simulink model "sys10m_pss"  (Simulink 8.7)
settings: Solver=ode3  StartTime=0.0  StopTime=10  FixedStep=1e-2  MaxStep=1e-2  RelTol=1e-5
values from neighbouring files (symbols this model uses):
  Kpss1 = KG1*T11*T13/(T12*T14)    [initSSA.m]    (also in pss_objf.m)
  Kpss10 = KG10*T101*T103/(T102*T104)    [initSSA.m]    (also in pss_objf.m)
  Kpss3 = KG3*T31*T33/(T32*T34)    [initSSA.m]    (also in pss_objf.m)
  Kpss4 = KG4*T41*T43/(T42*T44)    [initSSA.m]    (also in pss_objf.m)
  Kpss5 = KG5*T51*T53/(T52*T54)    [initSSA.m]    (also in pss_objf.m)
  Kpss6 = KG6*T61*T63/(T62*T64)    [initSSA.m]    (also in pss_objf.m)
  Kpss7 = KG7*T71*T73/(T72*T74)    [initSSA.m]    (also in pss_objf.m)
  Kpss8 = KG8*T81*T83/(T82*T84)    [initSSA.m]    (also in pss_objf.m)
  Kpss9 = KG9*T91*T93/(T92*T94)    [initSSA.m]    (also in pss_objf.m)
  T101 = x(42)    [initSSA.m]    (also in pss_objf.m)
  T102 = x(43)    [initSSA.m]    (also in pss_objf.m)
  T103 = x(44)    [initSSA.m]    (also in pss_objf.m)
  T104 = x(45)    [initSSA.m]    (also in pss_objf.m)
  T11 = x(10)    [initSSA.m]    (also in pss_objf.m)
  T12 = x(11)    [initSSA.m]    (also in pss_objf.m)
  T13 = x(12)    [initSSA.m]    (also in pss_objf.m)
  T14 = x(13)    [initSSA.m]    (also in pss_objf.m)
  T31 = x(14)    [initSSA.m]    (also in pss_objf.m)
  T32 = x(15)    [initSSA.m]    (also in pss_objf.m)
  T33 = x(16)    [initSSA.m]    (also in pss_objf.m)
  T34 = x(17)    [initSSA.m]    (also in pss_objf.m)
  T41 = x(18)    [initSSA.m]    (also in pss_objf.m)
  T42 = x(19)    [initSSA.m]    (also in pss_objf.m)
  T43 = x(20)    [initSSA.m]    (also in pss_objf.m)
  T44 = x(21)    [initSSA.m]    (also in pss_objf.m)
  T51 = x(22)    [initSSA.m]    (also in pss_objf.m)
  T52 = x(23)    [initSSA.m]    (also in pss_objf.m)
  T53 = x(24)    [initSSA.m]    (also in pss_objf.m)
  T54 = x(25)    [initSSA.m]    (also in pss_objf.m)
  T61 = x(26)    [initSSA.m]    (also in pss_objf.m)
  T62 = x(27)    [initSSA.m]    (also in pss_objf.m)
  T63 = x(28)    [initSSA.m]    (also in pss_objf.m)
  T64 = x(29)    [initSSA.m]    (also in pss_objf.m)
  T71 = x(30)    [initSSA.m]    (also in pss_objf.m)
  T72 = x(31)    [initSSA.m]    (also in pss_objf.m)
  T73 = x(32)    [initSSA.m]    (also in pss_objf.m)
  T74 = x(33)    [initSSA.m]    (also in pss_objf.m)
  T81 = x(34)    [initSSA.m]    (also in pss_objf.m)
  T82 = x(35)    [initSSA.m]    (also in pss_objf.m)
  T83 = x(36)    [initSSA.m]    (also in pss_objf.m)
  T84 = x(37)    [initSSA.m]    (also in pss_objf.m)
  T91 = x(38)    [initSSA.m]    (also in pss_objf.m)
  T92 = x(39)    [initSSA.m]    (also in pss_objf.m)
  T93 = x(40)    [initSSA.m]    (also in pss_objf.m)
  T94 = x(41)    [initSSA.m]    (also in pss_objf.m)
  Tw = 10    [initSSA.m]    (also in pss_objf.m)
undefined symbols (not defined in the file or in its folder): D, delta0, Efd0, Epd0, Epq0, event, fYred, KA, M, m, small_d, TA, Tpd0, Tpq0, Vref1, ws, XXdpd, XXpdq, XXqpq, Yred, Zdq
libraries: powerlib_extras x2
settings Model: Creator=hbeiran  LastModifiedBy=EBUKA
settings SolverCC: AlgebraicLoopSolver=LineSearch
settings DataIOCC: LimitDataPoints=off  SignalLoggingSaveFormat=ModelDataLogs
settings OptimizationCC: DefaultParameterBehavior=Inlined  BufferReuse=off  ExpressionDepthLimit=2147483647
settings DebuggingCC: AlgebraicLoopMsg=none  SolverPrmCheckMsg=warning  FcnCallInpInsideContextMsg=UseLocalSettings  StateNameClashWarn=warning  InitInArrayFormatMsg=none
settings SFSimCC: SimParseCustomCode=off
settings GRTTargetCC: CombineOutputUpdateFcns=off  GRTInterface=on
settings ConfigurationSet: Description=SimMechanics 2G

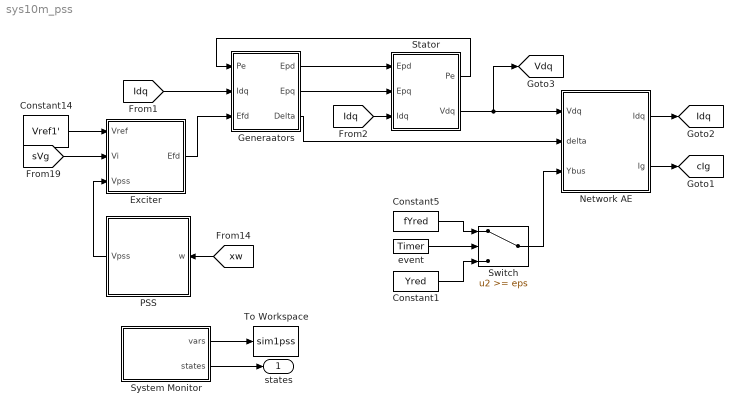
== system sys10m_pss ==
  Constant1 : Constant  Value=Yred  VectorParams1D=off
  Constant14 : Constant  Value=Vref1'  VectorParams1D=off
  Constant5 : Constant  Value=fYred  VectorParams1D=off
  Exciter : Subsystem
  Generaators : Subsystem
  Network AE : MATLAB Function  TreatAsAtomicUnit=on
  PSS : Subsystem
  Stator : Subsystem
  Switch : Switch  Threshold=eps
  System Monitor : Subsystem
  To Workspace : ToWorkspace  VariableName=sim1pss  SaveFormat=Structure With Time  SampleTime=-1
  event : powerlib_extras/Control  Blocks/Timer  t=event(1,:)  e=event(2,:)
  states : Outport
  tag scope: Idq=global, Vdq=global, cIg=global
  wires:
  Exciter/1(Efd) -> Generaators/3(Efd)
  Constant14/1 -> Exciter/1(Vref)
  [Idq] -> Generaators/2(Idq)
  Network AE/1(Idq) -> [Idq]
  event/1 -> Switch/2
  Constant5/1 -> Switch/1
  Constant1/1 -> Switch/3
  Switch/1 -> Network AE/3(Ybus)
  System Monitor/1(vars) -> To Workspace/1
  System Monitor/2(states) -> states/1
  Generaators/3(Delta) -> Network AE/2(delta)
  Network AE/2(Ig) -> [cIg]
  Stator/2(Vdq) -> Network AE/1(Vdq), [Vdq]
  [Idq] -> Stator/3(Idq)
  Generaators/1(Epd) -> Stator/1(Epd)
  Generaators/2(Epq) -> Stator/2(Epq)
  Stator/1(Pe) -> Generaators/1(Pe)
  [sVg] -> Exciter/2(Vi)
  PSS/1(Vpss) -> Exciter/3(Vpss)
  [xw] -> PSS/1(w)

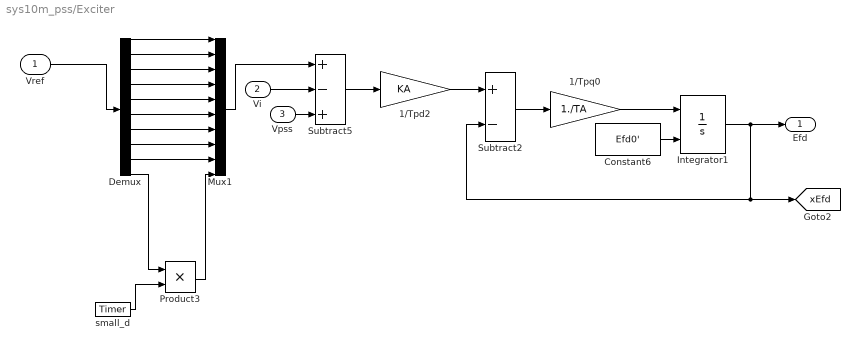
== system sys10m_pss/Exciter ==
  Vref : Inport
  Vi : Inport  Port=2
  Vpss : Inport  Port=3
  1/Tpd2 : Gain  Gain=KA
  1/Tpq0 : Gain  Gain=1./TA
  Constant6 : Constant  Value=Efd0'  VectorParams1D=off
  Demux : Demux  Outputs=10
  Integrator1 : Integrator  InitialConditionSource=external
  Mux1 : Mux  Inputs=10
  Product3 : Product  RndMeth=Zero
  Subtract2 : Sum  Inputs=+-
  Subtract5 : Sum  Inputs=+-+
  small_d : powerlib_extras/Control  Blocks/Timer  t=small_d(1,:)  e=small_d(2,:)
  Efd : Outport
  tag scope: xEfd=global
  wires:
  Constant6/1 -> Integrator1/2
  Subtract2/1 -> 1/Tpq0/1
  1/Tpq0/1 -> Integrator1/1
  Integrator1/1 -> Efd/1, Subtract2/2, [xEfd]
  Vi/1 -> Subtract5/2
  Subtract5/1 -> 1/Tpd2/1
  1/Tpd2/1 -> Subtract2/1
  Demux/1 -> Mux1/1
  Demux/2 -> Mux1/2
  small_d/1 -> Product3/2
  Mux1/1 -> Subtract5/1
  Vref/1 -> Demux/1
  Vpss/1 -> Subtract5/3
  Demux/3 -> Mux1/3
  Demux/4 -> Mux1/4
  Demux/5 -> Mux1/5
  Demux/6 -> Mux1/6
  Demux/7 -> Mux1/7
  Demux/8 -> Mux1/8
  Demux/9 -> Mux1/9
  Demux/10 -> Product3/1
  Product3/1 -> Mux1/10

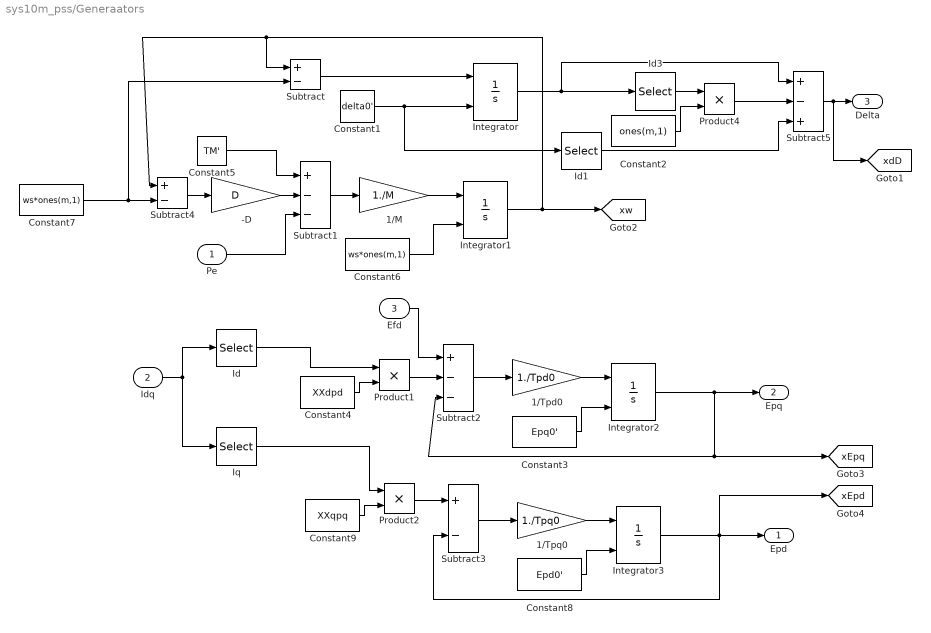
== system sys10m_pss/Generaators ==
  Pe : Inport
  Idq : Inport  Port=2
  Efd : Inport  Port=3
  -D : Gain  Gain=D
  1/M : Gain  Gain=1./M
  1/Tpd0 : Gain  Gain=1./Tpd0
  1/Tpq0 : Gain  Gain=1./Tpq0
  Constant1 : Constant  Value=delta0'  VectorParams1D=off
  Constant2 : Constant  Value=ones(m,1)  VectorParams1D=off
  Constant3 : Constant  Value=Epq0'  VectorParams1D=off
  Constant4 : Constant  Value=XXdpd  VectorParams1D=off
  Constant5 : Constant  Value=TM'  VectorParams1D=off
  Constant6 : Constant  Value=ws*ones(m,1)  VectorParams1D=off
  Constant7 : Constant  Value=ws*ones(m,1)  VectorParams1D=off
  Constant8 : Constant  Value=Epd0'  VectorParams1D=off
  Constant9 : Constant  Value=XXqpq  VectorParams1D=off
  Id : Selector  InputPortWidth=2*m  IndexOptions=Index vector (dialog)  Indices=[1:m]  OutputSizes=1
  Id1 : Selector  InputPortWidth=m  IndexOptions=Index vector (dialog)  Indices=[1]  OutputSizes=1
  Id3 : Selector  InputPortWidth=m  IndexOptions=Index vector (dialog)  Indices=[1]  OutputSizes=1
  Integrator{,1..3} (4 alike) : Integrator  InitialConditionSource=external
  Iq : Selector  InputPortWidth=2*m  IndexOptions=Index vector (dialog)  Indices=[m+1:2*m]  OutputSizes=1
  Product1 : Product  RndMeth=Zero
  Product2 : Product  RndMeth=Zero
  Product4 : Product  RndMeth=Zero
  Subtract : Sum  Inputs=+-
  Subtract1 : Sum  Inputs=+--
  Subtract2 : Sum  Inputs=+--
  Subtract3 : Sum  Inputs=+-
  Subtract4 : Sum  Inputs=+-
  Subtract5 : Sum  Inputs=+-+
  Epd : Outport
  Epq : Outport  Port=2
  Delta : Outport  Port=3
  tag scope: xEpd=global, xEpq=global, xdD=global, xw=global
  wires:
  Subtract/1 -> Integrator/1
  Constant5/1 -> Subtract1/1
  Subtract1/1 -> 1/M/1
  1/M/1 -> Integrator1/1
  Constant6/1 -> Integrator1/2
  -D/1 -> Subtract1/2
  Constant3/1 -> Integrator2/2
  Subtract2/1 -> 1/Tpd0/1
  Integrator2/1 -> Epq/1, Subtract2/3, [xEpq]
  Product1/1 -> Subtract2/2
  Constant4/1 -> Product1/2
  1/Tpd0/1 -> Integrator2/1
  Constant8/1 -> Integrator3/2
  Subtract3/1 -> 1/Tpq0/1
  Integrator3/1 -> Epd/1, [xEpd], Subtract3/2
  Constant9/1 -> Product2/2
  1/Tpq0/1 -> Integrator3/1
  Product2/1 -> Subtract3/1
  Efd/1 -> Subtract2/1
  Integrator1/1 -> [xw], Subtract/1, Subtract4/1
  Id/1 -> Product1/1
  Idq/1 -> Id/1, Iq/1
  Iq/1 -> Product2/1
  Pe/1 -> Subtract1/3
  Subtract4/1 -> -D/1
  Constant7/1 -> Subtract4/2, Subtract/2
  Subtract5/1 -> Delta/1, [xdD]
  Constant1/1 -> Integrator/2, Id1/1
  Integrator/1 -> Subtract5/1, Id3/1
  Id3/1 -> Product4/1
  Constant2/1 -> Product4/2
  Product4/1 -> Subtract5/2
  Id1/1 -> Subtract5/3

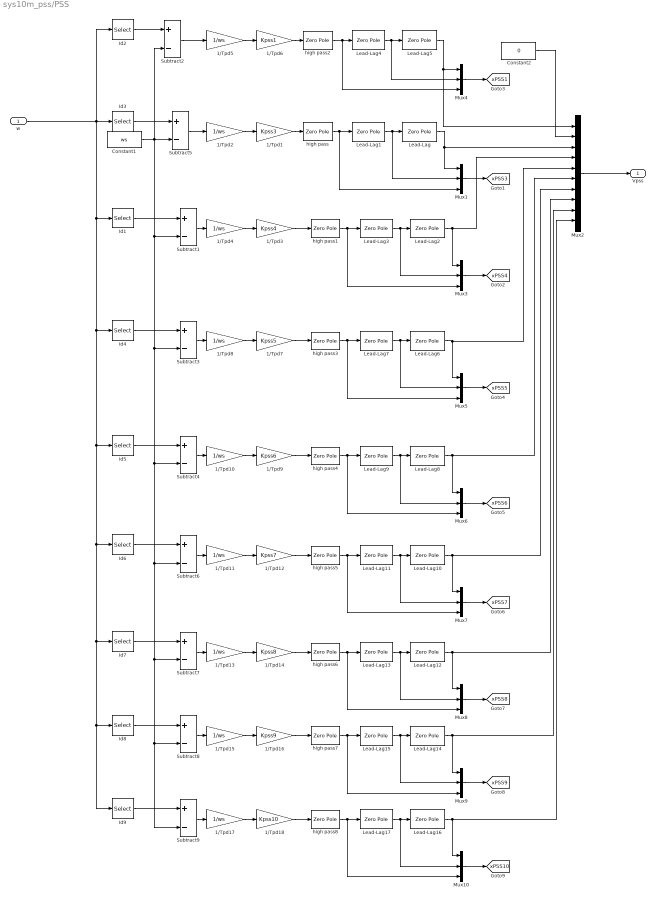
== system sys10m_pss/PSS ==
  w : Inport
  1/Tpd1 : Gain  Gain=Kpss3
  1/Tpd{2,4..5,8,10..11,13,15,17} (9 alike) : Gain  Gain=1/ws
  1/Tpd12 : Gain  Gain=Kpss7
  1/Tpd14 : Gain  Gain=Kpss8
  1/Tpd16 : Gain  Gain=Kpss9
  1/Tpd18 : Gain  Gain=Kpss10
  1/Tpd3 : Gain  Gain=Kpss4
  1/Tpd6 : Gain  Gain=Kpss1
  1/Tpd7 : Gain  Gain=Kpss5
  1/Tpd9 : Gain  Gain=Kpss6
  Constant1 : Constant  Value=ws  VectorParams1D=off
  Constant2 : Constant  Value=0  VectorParams1D=off
  Id1 : Selector  InputPortWidth=m  IndexOptions=Index vector (dialog)  Indices=[4]  OutputSizes=1
  Id2 : Selector  InputPortWidth=m  IndexOptions=Index vector (dialog)  Indices=[1]  OutputSizes=1
  Id3 : Selector  InputPortWidth=m  IndexOptions=Index vector (dialog)  Indices=[3]  OutputSizes=1
  Id4 : Selector  InputPortWidth=m  IndexOptions=Index vector (dialog)  Indices=[5]  OutputSizes=1
  Id5 : Selector  InputPortWidth=m  IndexOptions=Index vector (dialog)  Indices=[6]  OutputSizes=1
  Id6 : Selector  InputPortWidth=m  IndexOptions=Index vector (dialog)  Indices=[7]  OutputSizes=1
  Id7 : Selector  InputPortWidth=m  IndexOptions=Index vector (dialog)  Indices=[8]  OutputSizes=1
  Id8 : Selector  InputPortWidth=m  IndexOptions=Index vector (dialog)  Indices=[9]  OutputSizes=1
  Id9 : Selector  InputPortWidth=m  IndexOptions=Index vector (dialog)  Indices=[10]  OutputSizes=1
  Lead-Lag : ZeroPole  Zeros=[-1/T33]  Poles=[-1/T34]
  Lead-Lag1 : ZeroPole  Zeros=[-1/T31]  Poles=[-1/T32]
  Lead-Lag10 : ZeroPole  Zeros=[-1/T73]  Poles=[-1/T74]
  Lead-Lag11 : ZeroPole  Zeros=[-1/T71]  Poles=[-1/T72]
  Lead-Lag12 : ZeroPole  Zeros=[-1/T83]  Poles=[-1/T84]
  Lead-Lag13 : ZeroPole  Zeros=[-1/T81]  Poles=[-1/T82]
  Lead-Lag14 : ZeroPole  Zeros=[-1/T93]  Poles=[-1/T94]
  Lead-Lag15 : ZeroPole  Zeros=[-1/T91]  Poles=[-1/T92]
  Lead-Lag16 : ZeroPole  Zeros=[-1/T103]  Poles=[-1/T104]
  Lead-Lag17 : ZeroPole  Zeros=[-1/T101]  Poles=[-1/T102]
  Lead-Lag2 : ZeroPole  Zeros=[-1/T43]  Poles=[-1/T44]
  Lead-Lag3 : ZeroPole  Zeros=[-1/T41]  Poles=[-1/T42]
  Lead-Lag4 : ZeroPole  Zeros=[-1/T11]  Poles=[-1/T12]
  Lead-Lag5 : ZeroPole  Zeros=[-1/T13]  Poles=[-1/T14]
  Lead-Lag6 : ZeroPole  Zeros=[-1/T53]  Poles=[-1/T54]
  Lead-Lag7 : ZeroPole  Zeros=[-1/T51]  Poles=[-1/T52]
  Lead-Lag8 : ZeroPole  Zeros=[-1/T63]  Poles=[-1/T64]
  Lead-Lag9 : ZeroPole  Zeros=[-1/T61]  Poles=[-1/T62]
  Mux{1,3..10} (9 alike) : Mux  Inputs=3
  Mux2 : Mux  Inputs=10
  Subtract{1..9} (9 alike) : Sum  Inputs=+-
  high pass{,1..8} (9 alike) : ZeroPole  Zeros=[0]  Poles=[-1/Tw]
  Vpss : Outport
  tag scope: xPSS10=global, xPSS1=global, xPSS3=global, xPSS4=global, xPSS5=global, xPSS6=global, xPSS7=global, xPSS8=global, xPSS9=global
  wires:
  Subtract5/1 -> 1/Tpd2/1
  1/Tpd1/1 -> high pass/1
  Lead-Lag/1 -> Mux2/3, Mux1/1
  high pass/1 -> Lead-Lag1/1, Mux1/3
  Lead-Lag1/1 -> Lead-Lag/1, Mux1/2
  Mux1/1 -> [xPSS3]
  1/Tpd2/1 -> 1/Tpd1/1
  Mux2/1 -> Vpss/1
  Id3/1 -> Subtract5/1
  Subtract1/1 -> 1/Tpd4/1
  1/Tpd3/1 -> high pass1/1
  Lead-Lag2/1 -> Mux2/4, Mux3/1
  high pass1/1 -> Mux3/3, Lead-Lag3/1
  Lead-Lag3/1 -> Mux3/2, Lead-Lag2/1
  Mux3/1 -> [xPSS4]
  1/Tpd4/1 -> 1/Tpd3/1
  Id1/1 -> Subtract1/1
  Id2/1 -> Subtract2/1
  Subtract2/1 -> 1/Tpd5/1
  1/Tpd5/1 -> 1/Tpd6/1
  1/Tpd6/1 -> high pass2/1
  high pass2/1 -> Mux4/3, Lead-Lag4/1
  Lead-Lag4/1 -> Mux4/2, Lead-Lag5/1
  Lead-Lag5/1 -> Mux2/1, Mux4/1
  Mux4/1 -> [xPSS1]
  Subtract3/1 -> 1/Tpd8/1
  1/Tpd7/1 -> high pass3/1
  Lead-Lag6/1 -> Mux2/5, Mux5/1
  high pass3/1 -> Lead-Lag7/1, Mux5/3
  Lead-Lag7/1 -> Lead-Lag6/1, Mux5/2
  Mux5/1 -> [xPSS5]
  1/Tpd8/1 -> 1/Tpd7/1
  Id4/1 -> Subtract3/1
  w/1 -> Id2/1, Id3/1, Id6/1, Id8/1, Id9/1, Id7/1, Id5/1, Id4/1, Id1/1
  Subtract4/1 -> 1/Tpd10/1
  1/Tpd9/1 -> high pass4/1
  high pass4/1 -> Mux6/3, Lead-Lag9/1
  Lead-Lag9/1 -> Mux6/2, Lead-Lag8/1
  Mux6/1 -> [xPSS6]
  1/Tpd10/1 -> 1/Tpd9/1
  Id5/1 -> Subtract4/1
  Subtract6/1 -> 1/Tpd11/1
  1/Tpd12/1 -> high pass5/1
  high pass5/1 -> Lead-Lag11/1, Mux7/3
  Lead-Lag11/1 -> Lead-Lag10/1, Mux7/2
  Mux7/1 -> [xPSS7]
  1/Tpd11/1 -> 1/Tpd12/1
  Id6/1 -> Subtract6/1
  Subtract7/1 -> 1/Tpd13/1
  1/Tpd14/1 -> high pass6/1
  high pass6/1 -> Mux8/3, Lead-Lag13/1
  Lead-Lag13/1 -> Mux8/2, Lead-Lag12/1
  Mux8/1 -> [xPSS8]
  1/Tpd13/1 -> 1/Tpd14/1
  Id7/1 -> Subtract7/1
  Lead-Lag8/1 -> Mux2/6, Mux6/1
  Lead-Lag10/1 -> Mux2/7, Mux7/1
  Lead-Lag12/1 -> Mux2/8, Mux8/1
  Subtract8/1 -> 1/Tpd15/1
  1/Tpd16/1 -> high pass7/1
  high pass7/1 -> Lead-Lag15/1, Mux9/3
  Lead-Lag15/1 -> Lead-Lag14/1, Mux9/2
  Mux9/1 -> [xPSS9]
  1/Tpd15/1 -> 1/Tpd16/1
  Id8/1 -> Subtract8/1
  Lead-Lag14/1 -> Mux2/9, Mux9/1
  Constant1/1 -> Subtract2/2, Subtract5/2, Subtract7/2, Subtract9/2, Subtract8/2, Subtract6/2, Subtract4/2, Subtract3/2, Subtract1/2
  Subtract9/1 -> 1/Tpd17/1
  1/Tpd18/1 -> high pass8/1
  high pass8/1 -> Mux10/3, Lead-Lag17/1
  Lead-Lag17/1 -> Mux10/2, Lead-Lag16/1
  Mux10/1 -> [xPSS10]
  1/Tpd17/1 -> 1/Tpd18/1
  Id9/1 -> Subtract9/1
  Lead-Lag16/1 -> Mux2/10, Mux10/1
  Constant2/1 -> Mux2/2

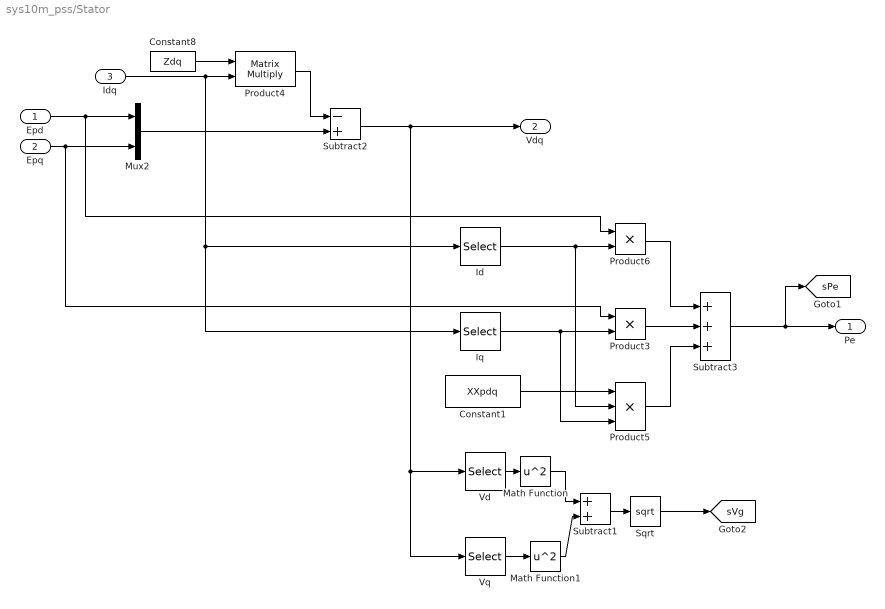
== system sys10m_pss/Stator ==
  Epd : Inport
  Epq : Inport  Port=2
  Idq : Inport  Port=3
  Constant1 : Constant  Value=XXpdq  VectorParams1D=off
  Constant8 : Constant  Value=Zdq  VectorParams1D=off
  Id : Selector  InputPortWidth=2*m  IndexOptions=Index vector (dialog)  Indices=[1:m]  OutputSizes=1
  Iq : Selector  InputPortWidth=2*m  IndexOptions=Index vector (dialog)  Indices=[m+1:2*m]  OutputSizes=1
  Math Function : Math  Operator=square  SaturateOnIntegerOverflow=on
  Math Function1 : Math  Operator=square  SaturateOnIntegerOverflow=on
  Mux2 : Mux  Inputs=2
  Product3 : Product  RndMeth=Zero
  Product4 : Product  Multiplication=Matrix(*)  RndMeth=Zero
  Product5 : Product  Inputs=3  RndMeth=Zero
  Product6 : Product  RndMeth=Zero
  Sqrt : Sqrt  SaturateOnIntegerOverflow=on
  Subtract1 : Sum
  Subtract2 : Sum  Inputs=-+
  Subtract3 : Sum  Inputs=+++
  Vd : Selector  InputPortWidth=2*m  IndexOptions=Index vector (dialog)  Indices=[1:m]  OutputSizes=1
  Vq : Selector  InputPortWidth=2*m  IndexOptions=Index vector (dialog)  Indices=[m+1:2*m]  OutputSizes=1
  Pe : Outport
  Vdq : Outport  Port=2
  tag scope: sPe=global, sVg=global
  wires:
  Constant8/1 -> Product4/1
  Epd/1 -> Mux2/1, Product6/1
  Epq/1 -> Product3/1, Mux2/2
  Iq/1 -> Product5/3, Product3/2
  Product6/1 -> Subtract3/1
  Product3/1 -> Subtract3/2
  Product5/1 -> Subtract3/3
  Constant1/1 -> Product5/1
  Subtract3/1 -> Pe/1, [sPe]
  Id/1 -> Product6/2, Product5/2
  Vd/1 -> Math Function/1
  Vq/1 -> Math Function1/1
  Math Function/1 -> Subtract1/1
  Math Function1/1 -> Subtract1/2
  Subtract1/1 -> Sqrt/1
  Sqrt/1 -> [sVg]
  Mux2/1 -> Subtract2/2
  Idq/1 -> Product4/2, Id/1, Iq/1
  Product4/1 -> Subtract2/1
  Subtract2/1 -> Vdq/1, Vq/1, Vd/1

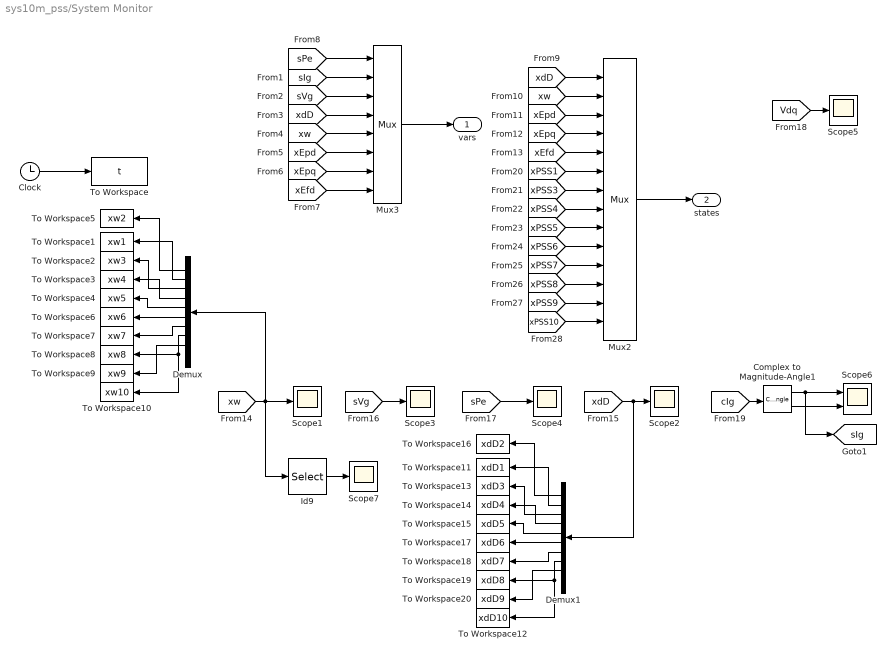
== system sys10m_pss/System Monitor ==
  Clock : Clock
  Complex to Magnitude-Angle1 : ComplexToMagnitudeAngle
  Demux : Demux  Outputs=10
  Demux1 : Demux  Outputs=10
  Id9 : Selector  InputPortWidth=m  IndexOptions=Index vector (dialog)  Indices=[1]  OutputSizes=1
  Mux2 : Mux  Inputs=14
  Mux3 : Mux  Inputs=8
  Scope{1..5,7} (6 alike) : Scope
  Scope6 : Scope  NumInputPorts=2
  To Workspace : ToWorkspace  VariableName=t  SampleTime=-1
      settings: Save2DSignal=2-D array (concatenate along first dimension)
  To Workspace1 : ToWorkspace  VariableName=xw1  SampleTime=-1
      settings: Save2DSignal=2-D array (concatenate along first dimension)
  To Workspace10 : ToWorkspace  VariableName=xw10  SampleTime=-1
      settings: Save2DSignal=2-D array (concatenate along first dimension)
  To Workspace11 : ToWorkspace  VariableName=xdD1  SampleTime=-1
      settings: Save2DSignal=2-D array (concatenate along first dimension)
  To Workspace12 : ToWorkspace  VariableName=xdD10  SampleTime=-1
      settings: Save2DSignal=2-D array (concatenate along first dimension)
  To Workspace13 : ToWorkspace  VariableName=xdD3  SampleTime=-1
      settings: Save2DSignal=2-D array (concatenate along first dimension)
  To Workspace14 : ToWorkspace  VariableName=xdD4  SampleTime=-1
      settings: Save2DSignal=2-D array (concatenate along first dimension)
  To Workspace15 : ToWorkspace  VariableName=xdD5  SampleTime=-1
      settings: Save2DSignal=2-D array (concatenate along first dimension)
  To Workspace16 : ToWorkspace  VariableName=xdD2  SampleTime=-1
      settings: Save2DSignal=2-D array (concatenate along first dimension)
  To Workspace17 : ToWorkspace  VariableName=xdD6  SampleTime=-1
      settings: Save2DSignal=2-D array (concatenate along first dimension)
  To Workspace18 : ToWorkspace  VariableName=xdD7  SampleTime=-1
      settings: Save2DSignal=2-D array (concatenate along first dimension)
  To Workspace19 : ToWorkspace  VariableName=xdD8  SampleTime=-1
      settings: Save2DSignal=2-D array (concatenate along first dimension)
  To Workspace2 : ToWorkspace  VariableName=xw3  SampleTime=-1
      settings: Save2DSignal=2-D array (concatenate along first dimension)
  To Workspace20 : ToWorkspace  VariableName=xdD9  SampleTime=-1
      settings: Save2DSignal=2-D array (concatenate along first dimension)
  To Workspace3 : ToWorkspace  VariableName=xw4  SampleTime=-1
      settings: Save2DSignal=2-D array (concatenate along first dimension)
  To Workspace4 : ToWorkspace  VariableName=xw5  SampleTime=-1
      settings: Save2DSignal=2-D array (concatenate along first dimension)
  To Workspace5 : ToWorkspace  VariableName=xw2  SampleTime=-1
      settings: Save2DSignal=2-D array (concatenate along first dimension)
  To Workspace6 : ToWorkspace  VariableName=xw6  SampleTime=-1
      settings: Save2DSignal=2-D array (concatenate along first dimension)
  To Workspace7 : ToWorkspace  VariableName=xw7  SampleTime=-1
      settings: Save2DSignal=2-D array (concatenate along first dimension)
  To Workspace8 : ToWorkspace  VariableName=xw8  SampleTime=-1
      settings: Save2DSignal=2-D array (concatenate along first dimension)
  To Workspace9 : ToWorkspace  VariableName=xw9  SampleTime=-1
      settings: Save2DSignal=2-D array (concatenate along first dimension)
  vars : Outport
  states : Outport  Port=2
  tag scope: sIg=global
  wires:
  Mux3/1 -> vars/1
  [sPe] -> Mux3/1
  [sIg] -> Mux3/2
  [sVg] -> Mux3/3
  [xdD] -> Mux3/4
  [xw] -> Mux3/5
  [xEpd] -> Mux3/6
  [xEpq] -> Mux3/7
  [xEfd] -> Mux3/8
  [xw] -> Mux2/2
  [xEpd] -> Mux2/3
  [xEpq] -> Mux2/4
  [xEfd] -> Mux2/5
  [xdD] -> Mux2/1
  Mux2/1 -> states/1
  [xw] -> Demux/1, Id9/1, Scope1/1
  [xdD] -> Demux1/1, Scope2/1
  [sVg] -> Scope3/1
  [sPe] -> Scope4/1
  Complex to Magnitude-Angle1/1 -> Scope6/1, [sIg]
  Complex to Magnitude-Angle1/2 -> Scope6/2
  [cIg] -> Complex to Magnitude-Angle1/1
  [Vdq] -> Scope5/1
  [xPSS1] -> Mux2/6
  [xPSS3] -> Mux2/7
  [xPSS4] -> Mux2/8
  [xPSS5] -> Mux2/9
  [xPSS6] -> Mux2/10
  [xPSS7] -> Mux2/11
  [xPSS8] -> Mux2/12
  [xPSS10] -> Mux2/14
  [xPSS9] -> Mux2/13
  Id9/1 -> Scope7/1
  Clock/1 -> To Workspace/1
  Demux/1 -> To Workspace5/1
  Demux/2 -> To Workspace1/1
  Demux/3 -> To Workspace2/1
  Demux/4 -> To Workspace3/1
  Demux/5 -> To Workspace4/1
  Demux/6 -> To Workspace6/1
  Demux/7 -> To Workspace7/1
  Demux/8 -> To Workspace10/1, To Workspace8/1
  Demux/9 -> To Workspace9/1
  Demux1/1 -> To Workspace16/1
  Demux1/2 -> To Workspace11/1
  Demux1/3 -> To Workspace13/1
  Demux1/4 -> To Workspace14/1
  Demux1/5 -> To Workspace15/1
  Demux1/6 -> To Workspace17/1
  Demux1/7 -> To Workspace18/1
  Demux1/8 -> To Workspace12/1, To Workspace19/1
  Demux1/9 -> To Workspace20/1

== matlab function Network AE ==
  data: Vdq input double; Idq output double; delta input double; Ig output double; Ybus input double
function [Idq, Ig] = fcn(Vdq,delta,Ybus)
%#codegen
% global_var

% Idq

Tm = diag(exp(1j*(delta-pi/2)));
iTm = diag(exp(-1j*(delta-pi/2)));
% iTm = inv(Tm);
% Tm=eye(3);
Vg = Tm*(Vdq(1:10,1)+1j*Vdq(11:20,1));
% VLoad=VL(4:9,1);
% Vbus=[Vg;VLoad];


I = Ybus*Vg;
Ig=I(1:10,1);
Id=real(iTm*Ig);
Iq=imag(iTm*Ig);

Idq=[Id;Iq];
